simulink model "modulator_3rd_order"  (Simulink 7.6)
settings: Solver=FixedStepDiscrete  StartTime=0.0  StopTime=9  RelTol=1e-3
settings Model: Creator=donze  LastModifiedBy=srirams  ExtModeAutoUpdateStatusClock=off
settings DataIOCC: LimitDataPoints=off  SaveFinalState=on  SaveState=on  SignalLoggingName=sigsOut
settings OptimizationCC: InlineInvariantSignals=on  InitFltsAndDblsToZero=on
settings DebuggingCC: SaveWithParameterizedLinksMsg=none  SignalResolutionControl=TryResolveAllWithWarning  SolverPrmCheckMsg=none  MultiTaskDSMMsg=warning  MultiTaskCondExecSysMsg=none  InitInArrayFormatMsg=none  StrictBusMsg=None
settings HardwareCC: TargetBitPerLong=64  TargetBitPerPointer=64  TargetEndianess=LittleEndian  TargetWordSize=64  TargetHWDeviceType=MATLAB Host  ProdEqTarget=off
settings RTWCC: SystemTargetFile=rsim.tlc  TemplateMakefile=rsim_default_tmf  Description=Rapid Simulation Target  ProcessScript=rsim_make_rtw_hook  IncludeERTFirstTime=on
settings RSimTargetCC: TargetFcnLib=ansi_tfl_tmw.mat  TargetFunctionLibrary=ANSI_C  ERTMultiwordTypeDef=System defined  ERTCodeCoverageTool=None  ERTMultiwordLength=256  IsPILTarget=off  EnableShiftOperators=on  PortableWordSizes=off

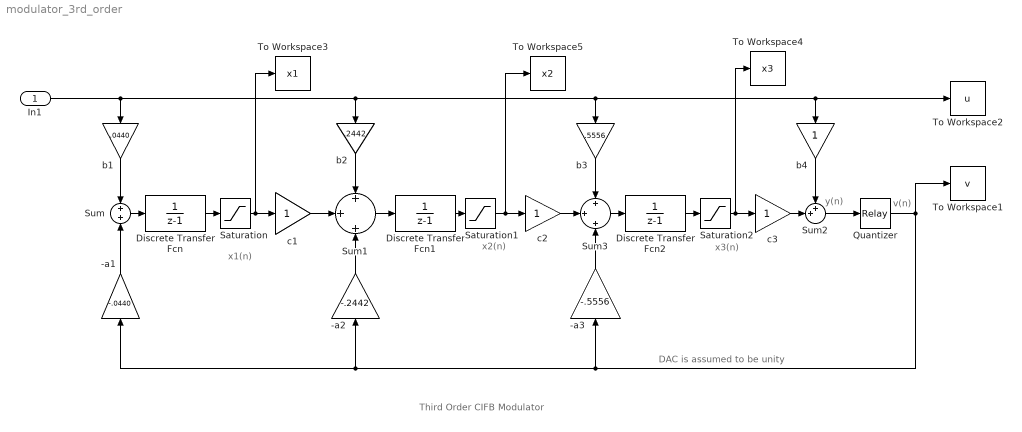
== system modulator_3rd_order ==
  note: x1(n)
  note: x2(n)
  note: x3(n)
  note: y(n)
  note: v(n)
  note: DAC is assumed to be unity
  note: Third Order CIFB Modulator
  In1 : Inport
  -a1 : Gain  Gain=-.0440  SaturateOnIntegerOverflow=on  OutDataTypeStr=Inherit: Same as input  ParamDataTypeStr=Inherit: Same as input
  -a2 : Gain  Gain=-.2442  SaturateOnIntegerOverflow=on  OutDataTypeStr=Inherit: Same as input  ParamDataTypeStr=Inherit: Same as input
  -a3 : Gain  Gain=-.5556  SaturateOnIntegerOverflow=on  OutDataTypeStr=Inherit: Same as input  ParamDataTypeStr=Inherit: Same as input
  Discrete Transfer Fcn : DiscreteTransferFcn  Denominator=[1 -1]  SampleTime=.05
  Discrete Transfer Fcn1 : DiscreteTransferFcn  Denominator=[1 -1]  SampleTime=.05
  Discrete Transfer Fcn2 : DiscreteTransferFcn  Denominator=[1 -1]  SampleTime=.05
  Quantizer : Relay  OffSwitchValue=-eps  OffOutputValue=-1
  Saturation : Saturate  UpperLimit=1  LowerLimit=-1  LinearizeAsGain=off
  Saturation1 : Saturate  UpperLimit=1  LowerLimit=-1
  Saturation2 : Saturate  UpperLimit=1  LowerLimit=-1
  Sum : Sum  SaturateOnIntegerOverflow=on
  Sum1 : Sum  Inputs=+|+|+  SaturateOnIntegerOverflow=on
  Sum2 : Sum  Inputs=++|  SaturateOnIntegerOverflow=on
  Sum3 : Sum  Inputs=+|+|+  SaturateOnIntegerOverflow=on
  To Workspace1 : ToWorkspace  VariableName=v  SampleTime=-1  SaveFormat=Array
  To Workspace2 : ToWorkspace  VariableName=u  SampleTime=-1  SaveFormat=Array
  To Workspace3 : ToWorkspace  VariableName=x1  SampleTime=-1  SaveFormat=Array
  To Workspace4 : ToWorkspace  VariableName=x3  SampleTime=-1  SaveFormat=Array
  To Workspace5 : ToWorkspace  VariableName=x2  SampleTime=-1  SaveFormat=Array
  b1 : Gain  Gain=.0440  SaturateOnIntegerOverflow=on  OutDataTypeStr=Inherit: Same as input  ParamDataTypeStr=Inherit: Same as input
  b2 : Gain  Gain=.2442  SaturateOnIntegerOverflow=on  OutDataTypeStr=Inherit: Same as input  ParamDataTypeStr=Inherit: Same as input
  b3 : Gain  Gain=.5556  SaturateOnIntegerOverflow=on  OutDataTypeStr=Inherit: Same as input  ParamDataTypeStr=Inherit: Same as input
  b4 : Gain  SaturateOnIntegerOverflow=on  OutDataTypeStr=Inherit: Same as input  ParamDataTypeStr=Inherit: Same as input
  c1 : Gain  SaturateOnIntegerOverflow=on  OutDataTypeStr=Inherit: Same as input  ParamDataTypeStr=Inherit: Same as input
  c2 : Gain  SaturateOnIntegerOverflow=on  OutDataTypeStr=Inherit: Same as input  ParamDataTypeStr=Inherit: Same as input
  c3 : Gain  SaturateOnIntegerOverflow=on  OutDataTypeStr=Inherit: Same as input  ParamDataTypeStr=Inherit: Same as input
  wires:
  Sum/1 -> Discrete Transfer Fcn/1
  -a1/1 -> Sum/2
  Sum1/1 -> Discrete Transfer Fcn1/1
  c2/1 -> Sum3/2
  b3/1 -> Sum3/1
  -a3/1 -> Sum3/3
  Sum3/1 -> Discrete Transfer Fcn2/1
  b4/1 -> Sum2/1
  b1/1 -> Sum/1
  Sum2/1 -> Quantizer/1
  Quantizer/1 -> -a3/1, -a1/1, -a2/1, To Workspace1/1
  c3/1 -> Sum2/2
  Discrete Transfer Fcn/1 -> Saturation/1
  Saturation/1 -> c1/1, To Workspace3/1
  Discrete Transfer Fcn1/1 -> Saturation1/1
  Saturation1/1 -> c2/1, To Workspace5/1
  Discrete Transfer Fcn2/1 -> Saturation2/1
  Saturation2/1 -> c3/1, To Workspace4/1
  b2/1 -> Sum1/1
  c1/1 -> Sum1/2
  -a2/1 -> Sum1/3
  In1/1 -> b1/1, b2/1, b3/1, b4/1, To Workspace2/1
